simulink model "H_Bridge_Microinverter_30KHz_2018a_16NOV18"  (R2018b)
settings: Solver=FixedStepDiscrete  StartTime=0.0  StopTime=3  RelTol=1e-3
undefined symbols (not defined in the file): sigbuilder_block
libraries: powerlib x43, powerlib_meascontrol x4, simulink x2, re_lib x1
settings Model: Creator=jasil  LastModifiedBy=jasil
settings DebuggingCC: LibraryContextMissingDiagnostic=none
settings CodeAppCC: StateflowObjectComments=on

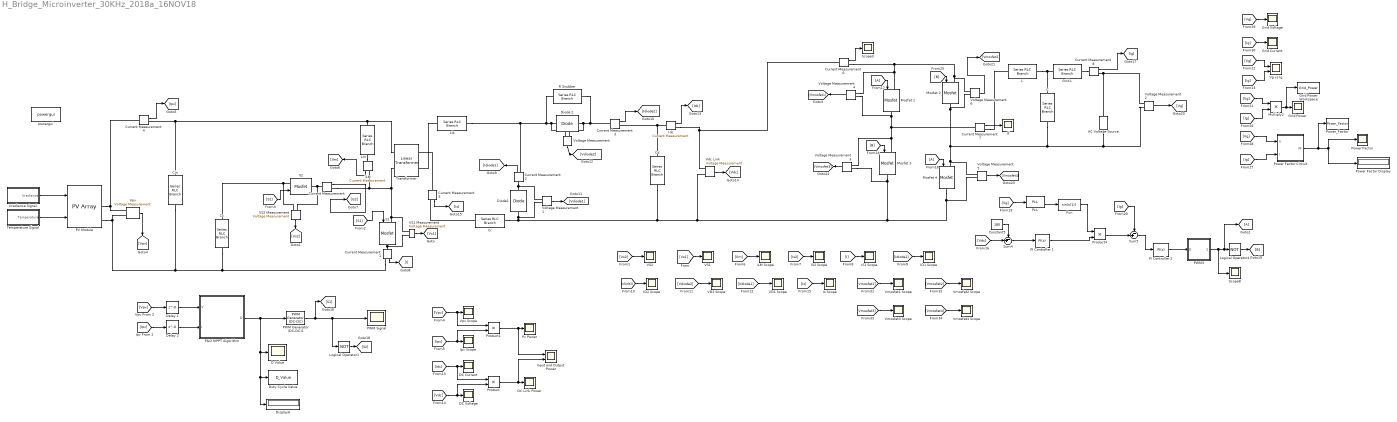
== system H_Bridge_Microinverter_30KHz_2018a_16NOV18 ==
  AC Voltage Source : powerlib/Electrical Sources/AC Voltage Source  Amplitude=120*sqrt(2)  Phase=0  Frequency=60  SampleTime=0  Measurements=None  BusType=swing  Pref=10e3  Qref=0  Qmin=-inf  Qmax=+inf
      settings: SourceProductName=Simscape Electrical
  C : powerlib/Elements/Series RLC Branch  LConnTagsString=__new0  RConnTagsString=__new0  BranchType=RC  Resistance=14.38  Inductance=1e-3  SetiL0=off  InitialCurrent=0  Capacitance=3.315727982e-5  Setx0=off  InitialVoltage=0  Measurements=None
      settings: SourceProductName=Simscape Electrical
  Cc : powerlib/Elements/Series RLC Branch  LConnTagsString=__new0  RConnTagsString=__new0  BranchType=RC  Resistance=0.000001  Inductance=1e-3  SetiL0=off  InitialCurrent=0  Capacitance=4e-6  Setx0=off  InitialVoltage=0  Measurements=None
      settings: SourceProductName=Simscape Electrical
  Cd : powerlib/Elements/Series RLC Branch  LConnTagsString=__new0  RConnTagsString=__new0  BranchType=RC  Resistance=0.000001  Inductance=1e-3  SetiL0=off  InitialCurrent=0  Capacitance=1e-3  Setx0=off  InitialVoltage=0  Measurements=None
      settings: SourceProductName=Simscape Electrical
  Cin : powerlib/Elements/Series RLC Branch  LConnTagsString=__new0  RConnTagsString=__new0  BranchType=RC  Resistance=0.000001  Inductance=1e-3  SetiL0=off  InitialCurrent=0  Capacitance=1e-3  Setx0=off  InitialVoltage=0  Measurements=Branch voltage
      settings: SourceProductName=Simscape Electrical
  Constant5 : Constant  Value=180
  Cr : powerlib/Elements/Series RLC Branch  LConnTagsString=__new0  RConnTagsString=__new0  BranchType=RC  Resistance=0.000001  Inductance=1e-3  SetiL0=off  InitialCurrent=0  Capacitance=2e-6  Setx0=off  InitialVoltage=0  Measurements=None
      settings: SourceProductName=Simscape Electrical
  Current Measurement{,1..8} (9 alike) : powerlib/Measurements/Current Measurement  PhasorSimulation=off  OutputType=Complex  PSBequivalent=0
      settings: SourceProductName=Simscape Electrical
  D Value : Scope
  DC Current : Scope
  DC Link Power : Scope
  DC Voltage : Scope
  Delay 1 : Delay  DelayLength=0  SampleTime=0.01
  Delay 2 : Delay  DelayLength=0  SampleTime=0.01
  Diode 2 : powerlib/Power Electronics/Diode  Ron=0.01  Lon=0  Vf=1.8  IC=0  UseSnubber=0  Rs=inf  Cs=0  Measurements=off
      settings: SourceProductName=Simscape Electrical
  Diode1 : powerlib/Power Electronics/Diode  Ron=0.01  Lon=0  Vf=1.8  IC=0  UseSnubber=0  Rs=inf  Cs=0  Measurements=off
      settings: SourceProductName=Simscape Electrical
  Display6 : Display
  Duty Cycle Value : ToWorkspace  VariableName=D_Value  SaveFormat=Timeseries  SampleTime=-1
  Fcn : Fcn  Expr=sin(u(1))
  "Grid Current " : Scope
  Grid L : powerlib/Elements/Series RLC Branch  LConnTagsString=__new0  RConnTagsString=__new0  BranchType=RL  Resistance=10e-3  Inductance=5.092958179e-6  SetiL0=off  InitialCurrent=0  Capacitance=1e-6  Setx0=off  InitialVoltage=0  Measurements=None
      settings: SourceProductName=Simscape Electrical
  Grid Power : Scope
  Grid Power Workspace : ToWorkspace  VariableName=Grid_Power  SaveFormat=Timeseries  SampleTime=-1
  Grid Voltage : Scope
  I dc : powerlib/Measurements/Current Measurement  PhasorSimulation=off  OutputType=Complex  PSBequivalent=0
      settings: SourceProductName=Simscape Electrical
  ID1 Scope : Scope
  ID2 Scope : Scope
  IS1 Scope : Scope
  IS2 Scope : Scope
  If : Scope
  Input and Output Power : Scope  NumInputPorts=2
  Ipv Scope : Scope
  "Irradiance Signal " : Subsystem  Tag=STV Subsys  LoadFcn=sigbuilder_block('load');  StartFcn=sigbuilder_block('start');  StopFcn=sigbuilder_block('stop');  ClipboardFcn=sigbuilder_block('clipboard');  mask(Sigbuilder block){tuvar=[0:10]}
      mask help: Simulink:masks:SigbuilderBlock_MD
      mask init:
      | if ~strcmp(get_param(bdroot(gcbh),'SimulationStatus'),'stopped') tuvar = sigbuilder_block('maskInit'); end
      settings: CopyFcn=sigbuilder_block('copy');  DeleteFcn=sigbuilder_block('delete');  ModelCloseFcn=sigbuilder_block('modelClose');  PreSaveFcn=sigbuilder_block('preSave');  PauseFcn=sigbuilder_block('pause');  ContinueFcn=sigbuilder_block('continue');  NameChangeFcn=sigbuilder_block('namechange');  OpenFcn=sigbuilder_block('open',[6 30 1012.5 447.75 ]);  CloseFcn=sigbuilder_block('close');
      mask Display: plot(0, 0, 100, 100,[2, 2, 32, 32, 2], [68, 8, 8, 68, 68],[32, 2], [38, 38], [32, 19, 2],[53, 60, 44], [32, 17, 17, 2],[16, 16, 31, 31]);txt = getActiveGroup(gcbh);text(2, 100, txt,'verticalAlignment', 'top');
  Is Scope : Scope
  L : powerlib/Elements/Series RLC Branch  LConnTagsString=__new0  RConnTagsString=__new0  BranchType=RL  Resistance=70e-3  Inductance=0.0282842712  SetiL0=off  InitialCurrent=0  Capacitance=1e-6  Setx0=off  InitialVoltage=0  Measurements=None
      settings: SourceProductName=Simscape Electrical
  Llk : powerlib/Elements/Series RLC Branch  LConnTagsString=__new0  RConnTagsString=__new0  BranchType=RL  Resistance=0.000001  Inductance=2.6e-6  SetiL0=off  InitialCurrent=0  Capacitance=1e-6  Setx0=off  InitialVoltage=0  Measurements=None
      settings: SourceProductName=Simscape Electrical
  Lm : powerlib/Elements/Series RLC Branch  LConnTagsString=__new0  RConnTagsString=__new0  BranchType=RL  Resistance=0.000001  Inductance=10e-6  SetiL0=off  InitialCurrent=0  Capacitance=1e-6  Setx0=off  InitialVoltage=0  Measurements=None
      settings: SourceProductName=Simscape Electrical
  Logical Operator1 : Logic  Operator=NOT  AllPortsSameDT=off  OutDataTypeStr=boolean
  Logical Operator4 : Logic  Operator=NOT  AllPortsSameDT=off  OutDataTypeStr=boolean
  Mosfet {1..4} (4 alike) : powerlib/Power Electronics/Mosfet  Ron=0.1  Lon=0  Rd=0.01  Vfd=0  IC=0  Rs=1e5  Cs=inf  Measurements=off
      settings: SourceProductName=Simscape Electrical
  Multiply2 : Product
  P&O MPPT Algorithm : MATLAB Function  TreatAsAtomicUnit=on
  PI Controller 1 : simulink/Continuous/PID Controller  Controller=PI  Form=Parallel  TimeDomain=Discrete-time  SampleTime=-1  IntegratorMethod=Forward Euler  FilterMethod=Forward Euler  ControllerParametersSource=internal  P=0.1  I=20  D=0  UseFilter=on  N=100  TunerSelectOption=Transfer Function Based (PID Tuner App)  InitialConditionSource=internal  InitialConditionForIntegrator=0  InitialConditionForFilter=0  DifferentiatorICPrevScaledInput=0  ExternalReset=none  TrackingMode=off  Kt=1  LimitOutput=off  UpperSaturationLimit=inf  LowerSaturationLimit=-inf  LinearizeAsGain=on  AntiWindupMode=none  Kb=1  POutMin=[]  POutMax=[]  IOutMin=[]  IOutMax=[]  DOutMin=[]  DOutMax=[]  NOutMin=[]  NOutMax=[]  SumOutMin=[]  SumOutMax=[]  SaturationOutMin=[]  SaturationOutMax=[]  PParamMin=[]  PParamMax=[]  IParamMin=[]  IParamMax=[]  DParamMin=[]  DParamMax=[]  NParamMin=[]  NParamMax=[]  KbParamMin=[]  KbParamMax=[]  KtParamMin=[]  KtParamMax=[]  KbOutMin=[]  KbOutMax=[]  KtOutMin=[]  KtOutMax=[]  IntegratorOutMin=[]  IntegratorOutMax=[]  FilterOutMin=[]  FilterOutMax=[]  SumI1OutMin=[]  SumI1OutMax=[]  SumI2OutMin=[]  SumI2OutMax=[]  SumI3OutMin=[]  SumI3OutMax=[]  SumI4OutMin=[]  SumI4OutMax=[]  SumDOutMin=[]  SumDOutMax=[]  DifferentiatorOutMin=[]  DifferentiatorOutMax=[]  FilterDiffOutCoefMin=[]  FilterDiffOutCoefMax=[]  ReciprocalOutMin=[]  ReciprocalOutMax=[]  SumDenOutMin=[]  SumDenOutMax=[]  SumNumOutMin=[]  SumNumOutMax=[]  DivideOutMin=[]  DivideOutMax=[]  IntegratorContinuousStateAttributes=''  IntegratorStateMustResolveToSignalObject=off  IntegratorRTWStateStorageClass=Auto  FilterContinuousStateAttributes=''  FilterStateMustResolveToSignalObject=off  FilterRTWStateStorageClass=Auto  ParallelPVariant=InternalParameters  IdealPVariant=Disabled  IVariant=InternalParameters  DVariant=Disabled  IntegratorVariant=Discrete  SatVariant=Disabled  AWVariant=Passthrough  PCopyVariant=Disabled  TRVariant=Disabled  FdbkBlocksVariant=Forward  IdealPFdbkVariant=Disabled  SatFdbkVariant=Disabled  DerivativeFilterVariant=Disabled  NVariant=Disabled  NCopyVariant=Disabled_SignalSpec  FilterICVariant=Disabled  IntegratorICVariant=InternalICs  ExternalResetVariant=Disabled  TRSumVariant=Passthrough  SumFdbkVariant=Disabled  SumVariant=Sum_PI
  PI Controller 2 : simulink/Continuous/PID Controller  Controller=PI  Form=Parallel  TimeDomain=Discrete-time  SampleTime=-1  IntegratorMethod=Forward Euler  FilterMethod=Forward Euler  ControllerParametersSource=internal  P=100  I=1000  D=0  UseFilter=on  N=100  TunerSelectOption=Transfer Function Based (PID Tuner App)  InitialConditionSource=internal  InitialConditionForIntegrator=0  InitialConditionForFilter=0  DifferentiatorICPrevScaledInput=0  ExternalReset=none  TrackingMode=off  Kt=1  LimitOutput=off  UpperSaturationLimit=inf  LowerSaturationLimit=-inf  LinearizeAsGain=on  AntiWindupMode=none  Kb=1  POutMin=[]  POutMax=[]  IOutMin=[]  IOutMax=[]  DOutMin=[]  DOutMax=[]  NOutMin=[]  NOutMax=[]  SumOutMin=[]  SumOutMax=[]  SaturationOutMin=[]  SaturationOutMax=[]  PParamMin=[]  PParamMax=[]  IParamMin=[]  IParamMax=[]  DParamMin=[]  DParamMax=[]  NParamMin=[]  NParamMax=[]  KbParamMin=[]  KbParamMax=[]  KtParamMin=[]  KtParamMax=[]  KbOutMin=[]  KbOutMax=[]  KtOutMin=[]  KtOutMax=[]  IntegratorOutMin=[]  IntegratorOutMax=[]  FilterOutMin=[]  FilterOutMax=[]  SumI1OutMin=[]  SumI1OutMax=[]  SumI2OutMin=[]  SumI2OutMax=[]  SumI3OutMin=[]  SumI3OutMax=[]  SumI4OutMin=[]  SumI4OutMax=[]  SumDOutMin=[]  SumDOutMax=[]  DifferentiatorOutMin=[]  DifferentiatorOutMax=[]  FilterDiffOutCoefMin=[]  FilterDiffOutCoefMax=[]  ReciprocalOutMin=[]  ReciprocalOutMax=[]  SumDenOutMin=[]  SumDenOutMax=[]  SumNumOutMin=[]  SumNumOutMax=[]  DivideOutMin=[]  DivideOutMax=[]  IntegratorContinuousStateAttributes=''  IntegratorStateMustResolveToSignalObject=off  IntegratorRTWStateStorageClass=Auto  FilterContinuousStateAttributes=''  FilterStateMustResolveToSignalObject=off  FilterRTWStateStorageClass=Auto  ParallelPVariant=InternalParameters  IdealPVariant=Disabled  IVariant=InternalParameters  DVariant=Disabled  IntegratorVariant=Discrete  SatVariant=Disabled  AWVariant=Passthrough  PCopyVariant=Disabled  TRVariant=Disabled  FdbkBlocksVariant=Forward  IdealPFdbkVariant=Disabled  SatFdbkVariant=Disabled  DerivativeFilterVariant=Disabled  NVariant=Disabled  NCopyVariant=Disabled_SignalSpec  FilterICVariant=Disabled  IntegratorICVariant=InternalICs  ExternalResetVariant=Disabled  TRSumVariant=Passthrough  SumFdbkVariant=Disabled  SumVariant=Sum_PI
  PLL : powerlib_meascontrol/PLL/PLL  Fmin=60  Par_Init=[0, 60]  ParK=[180, 3200, 1]  TcD=1e-4  MaxRateChangeFreq=12  FilterCutOffFreq=25  Ts=1e-6  AGC=on
      settings: SourceProductName=Simscape Electrical  SourceProductBaseCode=PS
  PV Module : re_lib/Solar/PV Array  Npar=1  Nser=1  PlotType=array @ 25 deg.C & specified irradiances  S_vec="[ 1000  500  100 ]"  Temp_C_vec="[ 45 25  ]"  ModuleName=User-defined  PlotWhenSelected=off  Pm=179.9805  Ncell=36  Voc=24.06  Isc=9.77  Vm=19.67  Im=9.15  beta_Voc_pc=-0.28  alpha_Isc_pc=+0.04  beta_Voc=-0.067368  alpha_Isc=0.003908  IL=9.8911  I0=1.3829e-11  nI=0.95443  Rsh=60.4787  Rs=0.18212  BAL=off  Tc=1e-6  Tfilter=5e-5
      settings: SourceProductName=Simscape Electrical
  PWM Generator (DC-DC)1 : powerlib_meascontrol/Pulse & Signal Generators/PWM Generator (DC-DC)  Fsw=50000  Ts=0
      settings: SourceProductName=Simscape Electrical
  PWM Signal : Scope
  PWM3 : Subsystem
  Power Factor : Scope
  Power Factor Circuit : Subsystem
  Power Factor Display : Display
  Power_Factor : ToWorkspace  VariableName=Power_Factor  SaveFormat=Timeseries  SampleTime=-1
  Product : Product
  Product1 : Product
  Product4 : Product
  Pv Power : Scope
  R Snubber : powerlib/Elements/Series RLC Branch  LConnTagsString=__new0  RConnTagsString=__new0  BranchType=R  Resistance=1e6  Inductance=1e-3  SetiL0=off  InitialCurrent=0  Capacitance=1e-6  Setx0=off  InitialVoltage=0  Measurements=None
      settings: SourceProductName=Simscape Electrical
  S1 : powerlib/Power Electronics/Mosfet  Ron=7e-3  Lon=0  Rd=0.01  Vfd=1.3  IC=0  Rs=1e6  Cs=inf  Measurements=off
      settings: SourceProductName=Simscape Electrical
  S2 : powerlib/Power Electronics/Mosfet  Ron=7e-3  Lon=0  Rd=0.01  Vfd=1.3  IC=0  Rs=1e5  Cs=inf  Measurements=off
      settings: SourceProductName=Simscape Electrical
  Scope3 : Scope
  Scope8 : Scope
  Sum4 : Sum  Inputs=-+|
  Sum5 : Sum  Inputs=-+|
  Temperature Signal : Subsystem  Tag=STV Subsys  LoadFcn=sigbuilder_block('load');  StartFcn=sigbuilder_block('start');  StopFcn=sigbuilder_block('stop');  ClipboardFcn=sigbuilder_block('clipboard');  mask(Sigbuilder block){tuvar=[0:10]}
      mask help: Simulink:masks:SigbuilderBlock_MD
      mask init:
      | if ~strcmp(get_param(bdroot(gcbh),'SimulationStatus'),'stopped') tuvar = sigbuilder_block('maskInit'); end
      settings: CopyFcn=sigbuilder_block('copy');  DeleteFcn=sigbuilder_block('delete');  ModelCloseFcn=sigbuilder_block('modelClose');  PreSaveFcn=sigbuilder_block('preSave');  PauseFcn=sigbuilder_block('pause');  ContinueFcn=sigbuilder_block('continue');  NameChangeFcn=sigbuilder_block('namechange');  OpenFcn=sigbuilder_block('open',[6 30 1012.5 447.75 ]);  CloseFcn=sigbuilder_block('close');
      mask Display: plot(0, 0, 100, 100,[2, 2, 32, 32, 2], [68, 8, 8, 68, 68],[32, 2], [38, 38], [32, 19, 2],[53, 60, 44], [32, 17, 17, 2],[16, 16, 31, 31]);txt = getActiveGroup(gcbh);text(2, 100, txt,'verticalAlignment', 'top');
  Transformer : powerlib/Elements/Linear Transformer  UNITS=SI  NominalPower=[ 25 100e3 ]  winding1=[6.36 0 0]  winding2=[26.87 0 0]  ThreeWindings=off  winding3=[3.15e+05 3.969e+07 6316.9]  RmLm=[1e6 Inf]  Measurements=None  DataType=on
      settings: SourceProductName=Simscape Electrical
  VD1 Scope : Scope
  VD2 Scope : Scope
  VS1 : Scope
  VS1 Measurement : powerlib/Measurements/Voltage Measurement  PhasorSimulation=off  OutputType=Complex  PSBequivalent=0
      settings: SourceProductName=Simscape Electrical
  VS2 : Scope
  VS2 Measurement : powerlib/Measurements/Voltage Measurement  PhasorSimulation=off  OutputType=Complex  PSBequivalent=0
      settings: SourceProductName=Simscape Electrical
  Vdc Link : powerlib/Measurements/Voltage Measurement  PhasorSimulation=off  OutputType=Complex  PSBequivalent=0
      settings: SourceProductName=Simscape Electrical
  Vg vs Ig : Scope  NumInputPorts=2
  Vmosfet1 Scope : Scope
  Vmosfet2 Scope : Scope
  Vmosfet3 Scope : Scope
  Vmosfet4 Scope : Scope
  Voltage Measurement{,1..6} (7 alike) : powerlib/Measurements/Voltage Measurement  PhasorSimulation=off  OutputType=Complex  PSBequivalent=0
      Voltage Measurement settings: SourceProductName=Simscape Electrical
      Voltage Measurement1 settings: SourceProductName=Simscape Electrical
      Voltage Measurement2 settings: SourceProductName=Simscape Electrical
  Vpv : powerlib/Measurements/Voltage Measurement  PhasorSimulation=off  OutputType=Complex  PSBequivalent=0
      settings: SourceProductName=Simscape Electrical
  Vpv Scope : Scope
  iLM : powerlib/Measurements/Current Measurement  PhasorSimulation=off  OutputType=Complex  PSBequivalent=0
      settings: SourceProductName=Simscape Electrical
  iLM Scope : Scope
  powergui : powerlib/powergui  Priority=1  SimulationMode=Discrete  SampleTime=1e-7  frequency=60  Iterations=50  frequencyindice=0  Pbase=100e6  ErrMax=1e-4  UnitsV=kV  UnitsW=MW  buscounter=0  FunctionMessages=off  echomessages=off  EnableUseOfTLC=off  CurrentSourceSwitches=off  DisableSnubberDevices=off  DisableRonSwitches=off  DisableVfSwitches=off  DisplayEquations=off  SolverType=Tustin/Backward Euler (TBE)  Interpol=off  ExternalGateDelay=off  methode=off  Ts=100  x0status=blocks  SPID=on  SwTol=0  HookPort=off  RestoreLinks=warning  ResistiveCurrentMeasurement=off  Frange=[0:2:500]  Ylog=off  Xlog=on  ShowGrid=off  save=off  variable=ZData  structure=0  ZoomFFT=off  StartTime=0.0  cycles=1  DisplayStyle=1  fundamental=60  FreqAxis=off  MaxFrequency=1000  frequencyindicesteady=1  RmsSteady=1  display=off
  wires:
  [Vdiode1] -> VD1 Scope/1
  "Irradiance Signal "/1(Irradiance) -> PV Module/1
  [Vdc] -> Product/2, DC Voltage/1
  VS2 Measurement/1 -> [Vs2]
  Current Measurement1/1 -> [I]
  Vpv/1 -> [Vpv]
  Voltage Measurement/1 -> [Vdiode2]
  Voltage Measurement1/1 -> [Vdiode1]
  [S2] -> S2/1
  Current Measurement2/1 -> [Idiode1]
  [Vdiode2] -> VD2 Scope/1
  [Idiode1] -> ID1 Scope/1
  [Vpv] -> Product1/1, Vpv Scope/1
  [Ipv] -> Product1/2, Ipv Scope/1
  Current Measurement/1 -> [Is2]
  [Vs1] -> VS1/1
  [S1] -> S1/1
  [I] -> IS1 Scope/1
  [Vs2] -> VS2/1
  iLM/1 -> [Ilm]
  Product/1 -> Input and Output Power/2, DC Link Power/1
  [Ilm] -> iLM Scope/1
  [Idiode2] -> ID2 Scope/1
  Product1/1 -> Input and Output Power/1, Pv Power/1
  [Is2] -> IS2 Scope/1
  VS1 Measurement/1 -> [Vs1]
  [Idc] -> Product/1, DC Current/1
  Temperature Signal/1(Temperature) -> PV Module/2
  [Is] -> Is Scope/1
  Current Measurement4/1 -> [Ipv]
  I dc/1 -> [Idc]
  Current Measurement3/1 -> [Idiode2]
  Current Measurement5/1 -> [Is]
  [A] -> Mosfet 4/1
  PI Controller 1/1 -> Product4/2
  Product4/1 -> Sum5/2
  Constant5/1 -> Sum4/1
  Voltage Measurement2/1 -> [Vg]
  Current Measurement8/1 -> [Ig]
  PLL/2 -> Fcn/1
  [A] -> Mosfet 1/1
  Current Measurement7/1 -> If/1
  Logical Operator4/1 -> [B]
  Current Measurement6/1 -> Scope3/1
  [B] -> Mosfet 3/1
  PI Controller 2/1 -> PWM3/1(D)
  Sum4/1 -> PI Controller 1/1
  PWM3/1(S) -> Scope8/1, [A], Logical Operator4/1
  Sum5/1 -> PI Controller 2/1
  [B] -> Mosfet 2/1
  P&O MPPT Algorithm/1(D) -> Display6/1, Duty Cycle Value/1, D Value/1, PWM Generator (DC-DC)1/1
  PWM Generator (DC-DC)1/1 -> [S1], Logical Operator1/1, PWM Signal/1
  Delay 1/1 -> P&O MPPT Algorithm/1(V)
  Delay 2/1 -> P&O MPPT Algorithm/2(I)
  [Vpv] -> Delay 1/1
  [Ipv] -> Delay 2/1
  Logical Operator1/1 -> [S2]
  [Vdc] -> Sum4/2
  [Ig] -> Sum5/1
  [Vg] -> PLL/1
  Fcn/1 -> Product4/1
  [Ig] -> Multiply2/2
  [Vg] -> Vg vs Ig/1
  Multiply2/1 -> Grid Power Workspace/1, Grid Power/1
  [Ig] -> Vg vs Ig/2
  [Vg] -> Multiply2/1
  Power Factor Circuit/1(PF) -> Power_Factor/1, Power Factor/1, Power Factor Display/1
  [Ig] -> Power Factor Circuit/2(I)
  [Vg] -> Power Factor Circuit/1(V)
  [Ig] -> "Grid Current "/1
  [Vg] -> Grid Voltage/1
  Vdc Link/1 -> [Vdc]
  Voltage Measurement6/1 -> [Vmosfet2]
  Voltage Measurement4/1 -> [Vmosfet1]
  Voltage Measurement3/1 -> [Vmosfet3]
  Voltage Measurement5/1 -> [Vmosfet4]
  [Vmosfet1] -> Vmosfet1 Scope/1
  [Vmosfet2] -> Vmosfet2 Scope/1
  [Vmosfet3] -> Vmosfet3 Scope/1
  [Vmosfet4] -> Vmosfet4 Scope/1
  connections:
  Current Measurement1/RConn1 -- Vpv/LConn2 -- PV Module/RConn2 -- Cin/RConn1 -- Cc/RConn1
  Llk/RConn1 -- R Snubber/LConn1 -- Voltage Measurement/LConn2 -- Diode 2/LConn1 -- Current Measurement2/RConn1
  VS1 Measurement/LConn2 -- Current Measurement1/LConn1 -- S1/RConn1
  S2/LConn1 -- VS2 Measurement/LConn1 -- Cc/LConn1
  iLM/RConn1 -- S1/LConn1 -- VS1 Measurement/LConn1 -- Transformer/LConn2 -- Current Measurement/RConn1
  Cd/LConn1 -- I dc/LConn1 -- Current Measurement3/RConn1
  S2/RConn1 -- VS2 Measurement/LConn2 -- Current Measurement/LConn1
  Lm/RConn1 -- iLM/LConn1
  Cr/LConn1 -- Current Measurement5/RConn1
  I dc/RConn1 -- Current Measurement6/LConn1 -- Vdc Link/LConn1
  Lm/LConn1 -- Cin/LConn1 -- Current Measurement4/RConn1 -- Transformer/LConn1
  PV Module/RConn1 -- Vpv/LConn1 -- Current Measurement4/LConn1
  Diode 2/RConn1 -- Voltage Measurement/LConn1 -- R Snubber/RConn1 -- Current Measurement3/LConn1
  Diode1/RConn1 -- Voltage Measurement1/LConn1 -- Current Measurement2/LConn1
  Mosfet 4/RConn1 -- Voltage Measurement5/LConn2 -- Voltage Measurement3/LConn2 -- Mosfet 3/RConn1 -- Vdc Link/LConn2 -- Cr/RConn1 -- Voltage Measurement1/LConn2 -- Diode1/LConn1 -- Cd/RConn1
  Mosfet 4/LConn1 -- Voltage Measurement6/LConn2 -- Mosfet 2/RConn1 -- C/RConn1 -- Voltage Measurement2/LConn2 -- AC Voltage Source/LConn1 -- Voltage Measurement5/LConn1
  Current Measurement7/LConn1 -- Voltage Measurement3/LConn1 -- Mosfet 3/LConn1 -- Voltage Measurement4/LConn2 -- Mosfet 1/RConn1
  Current Measurement6/RConn1 -- Voltage Measurement6/LConn1 -- Mosfet 2/LConn1 -- Voltage Measurement4/LConn1 -- Mosfet 1/LConn1
  L/RConn1 -- Grid L/LConn1 -- C/LConn1
  Current Measurement7/RConn1 -- L/LConn1
  Llk/LConn1 -- Transformer/RConn2
  Current Measurement5/LConn1 -- Transformer/RConn1
  Voltage Measurement2/LConn1 -- AC Voltage Source/RConn1 -- Current Measurement8/RConn1
  Grid L/RConn1 -- Current Measurement8/LConn1

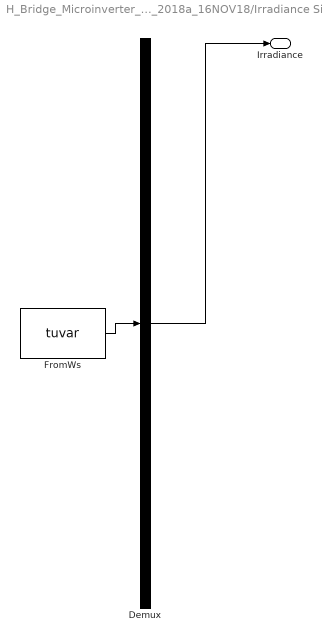
== system H_Bridge_Microinverter_30KHz_2018a_16NOV18/Irradiance Signal  ==
  Demux : Demux  Tag=STV Demux  Outputs=1
  FromWs : FromWorkspace  Tag=STV FromWs  VariableName=tuvar  SampleTime=0
      SigBuilderData=|
      | common.afterFinalStr = 'Extrapolate'
      | common.sampleTime = 0
      | dataSet.timeRange = [0 3]
      | dataSet.name = 'Group 1'
      | sbobj.Groups.Name = 'Group 1'
      | sbobj.Groups.Signals.Name = 'Irradiance'
      | sbobj.Groups.Signals.XData = [0 1 1 2 2 3]
      | sbobj.Groups.Signals.YData = [1250 1250 300 300 1100 1100]
      | sbobj.Groups.TimeRange = [0 3]
  Irradiance : Outport  Tag=STV Outport
  wires:
  Demux/1 -> Irradiance/1
  FromWs/1 -> Demux/1

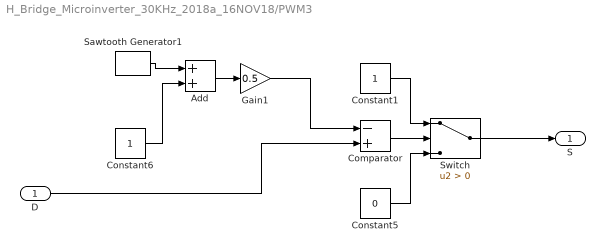
== system H_Bridge_Microinverter_30KHz_2018a_16NOV18/PWM3 ==
  D : Inport
  Add : Sum
  Comparator : Sum  Inputs=-+
  Constant1 : Constant
  Constant5 : Constant  Value=0
  Constant6 : Constant
  Gain1 : Gain  Gain=0.5
  Sawtooth Generator1 : powerlib_meascontrol/Pulse & Signal Generators/Sawtooth Generator  Freq=30000  Phase=180  Ts=0
      settings: SourceProductName=Simscape Electrical
  Switch : Switch  Criteria=u2 > Threshold
  S : Outport
  wires:
  Switch/1 -> S/1
  Constant1/1 -> Switch/1
  Comparator/1 -> Switch/2
  Constant6/1 -> Add/2
  Gain1/1 -> Comparator/1
  Constant5/1 -> Switch/3
  Sawtooth Generator1/1 -> Add/1
  Add/1 -> Gain1/1
  D/1 -> Comparator/2

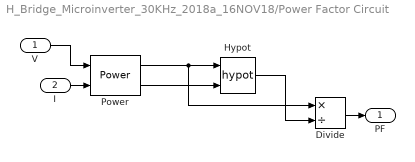
== system H_Bridge_Microinverter_30KHz_2018a_16NOV18/Power Factor Circuit ==
  V : Inport
  I : Inport  Port=2
  Divide : Product  Inputs=*/
  Hypot : Math  Operator=hypot  SaturateOnIntegerOverflow=on
  Power : powerlib_meascontrol/Measurements/Power  Freq=60  Vinit=[1, 0]  Iinit=[1, 0]  Ts=1e-6
      settings: SourceProductName=Simscape Power Systems
  PF : Outport
  wires:
  Divide/1 -> PF/1
  Hypot/1 -> Divide/2
  Power/1 -> Hypot/1, Divide/1
  I/1 -> Power/2
  V/1 -> Power/1
  Power/2 -> Hypot/2

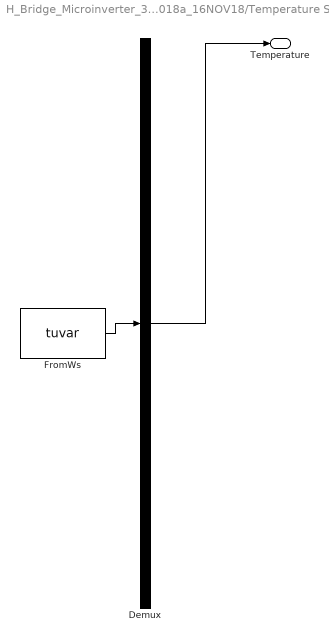
== system H_Bridge_Microinverter_30KHz_2018a_16NOV18/Temperature Signal ==
  Demux : Demux  Tag=STV Demux  Outputs=1
  FromWs : FromWorkspace  Tag=STV FromWs  VariableName=tuvar  SampleTime=0
      SigBuilderData=|
      | common.afterFinalStr = 'Extrapolate'
      | common.sampleTime = 0
      | dataSet.timeRange = [0 3]
      | dataSet.name = 'Group 1'
      | sbobj.Groups.Name = 'Group 1'
      | sbobj.Groups.Signals.Name = 'Temperature'
      | sbobj.Groups.Signals.XData = [0 1 1 2 2 3]
      | sbobj.Groups.Signals.YData = [25 25 75 75 50 50]
      | sbobj.Groups.TimeRange = [0 3]
  Temperature : Outport  Tag=STV Outport
  wires:
  Demux/1 -> Temperature/1
  FromWs/1 -> Demux/1

== matlab function H_Bridge_Microinverter_30KHz_2018a_16NOV18/P&O MPPT Algorithm ==
  data: V input; D output; I input
function D = PandO(V, I)
persistent p_prev;
persistent v_prev;
persistent d_prev; 


if isempty(d_prev)
    d_prev = 0.60;
    v_prev = 24.2;
    p_prev = 0;
end

% Select the change in duty cycle
delta_D = 0.01;

% Set local variables and calculate pv module power 
Vn = V;
In = I;
Pn = Vn*In;

% Increase or decrease duty cycle based on conditions
if ((Pn - p_prev) ~= 0)
    if ((Pn - p_prev) > 0)
        if ((Vn - v_prev) > 0)
            D = d_prev - delta_D;
        else
            D = d_prev + delta_D;
        end
    else
        if ((Vn - v_prev) > 0)
            D = d_prev + delta_D;
        else
            D = d_prev - delta_D;
        end        
    end
else
    D = d_prev;
end
% Update internal values
d_prev = D;
v_prev = Vn;
p_prev = Pn;
